simulink model "Dyn_Sim"  (Simulink 8.9)
settings: Solver=VariableStepAuto  StartTime=0.0  StopTime=time  FixedStep=0.1  MaxStep=0.1  RelTol=1e-3  EnableMultiTasking=on
values from neighbouring files (symbols this model uses):
  l1d = 2    [runner_simulation.m]
  l2d = 2    [runner_simulation.m]
  q0 = [gg gg 1]'.*[5 -4 pi/2]'    [runner_simulation.m]
  q0_1 = [gg gg 1]'.*[4 -6 pi/2]'    [runner_simulation.m]
  q0_2 = [gg gg 1]'.*[5 -6 pi/3]'    [runner_simulation.m]
  sai1_d = pi/2    (= 1.57079632679)    [runner_simulation.m]
  sai2_d = -pi/2    (= -1.57079632679)    [runner_simulation.m]
  u0 = [0.1;0.1;0.1]'    [runner_simulation.m]
  u01 = [0;0;0]'    [runner_simulation.m]
Description:
  | Real-Time Van der Pol Simulation
  | 
  | This demonstration shows a real-time version of the Simulink(R) Van der Pol
  | simulation demo. This model does not need any external signals, so it does
  | not need any data acquisition hardware or driver. This makes the model ideal
  | for first experiments with Real-Time Windows Target(TM), without need to
  | worry about proper I/O hardware configuration.
  | 
  | How to run this demo in Normal Mode:
  | 
  | 1) Double-click the orange button to switch to Normal Mode if needed.
  | 2) Start the real-time execution using Simulation->Start.
  | 3) Observe any missed ticks on the Missed Ticks scope.
  | 
  | How to run this demo in External Mode:
  | 
  | 1) Double-click the orange button to switch to External Mode if needed.
  | 2) Build the model using Tools->Code Generation->Build Model.
  | 3) Connect to the real-time code using Simulation->Connect to target.
  | 4) Start the real-time execution using Simulation->Start real-time code.
  | 5) Missed ticks will be always zero.
settings Model: Creator=The MathWorks Inc.  LastModifiedBy=Rasoul  ExtModeTrigDuration=101
settings DataIOCC: SignalLoggingSaveFormat=Dataset  SignalLoggingName=logsOut
settings OptimizationCC: ExpressionDepthLimit=2147483647  InitFltsAndDblsToZero=on  EfficientMapNaN2IntZero=off
settings DebuggingCC: SignalResolutionControl=TryResolveAllWithWarning  AllowSymbolicDim=off
settings HardwareCC: ProdBitPerPointer=64  ProdBitPerSizeT=64  ProdBitPerPtrDiffT=64  ProdLargestAtomicFloat=Float  ProdIntDivRoundTo=Zero  ProdEndianess=LittleEndian  ProdWordSize=64  ProdHWDeviceType=Intel->x86-64 (Windows64)  TargetBitPerLong=64  TargetBitPerPointer=64  TargetIntDivRoundTo=Zero  TargetEndianess=LittleEndian  TargetWordSize=64  TargetHWDeviceType=Intel->x86-64
settings RTWCC: SystemTargetFile=sldrt.tlc  TemplateMakefile=sldrt.tmf  Description=Simulink Desktop Real-Time  RTWCompilerOptimization=on
settings CodeAppCC: MaxIdLength=95
settings SimulinkDesktopRealTimeCC: TargetPreCompLibLocation=C:\Program Files\MATLAB\R2017a\toolbox\sldrt\lib\win64  TargetLangStandard=C89/C90 (ANSI)  SupportVariableSizeSignals=off

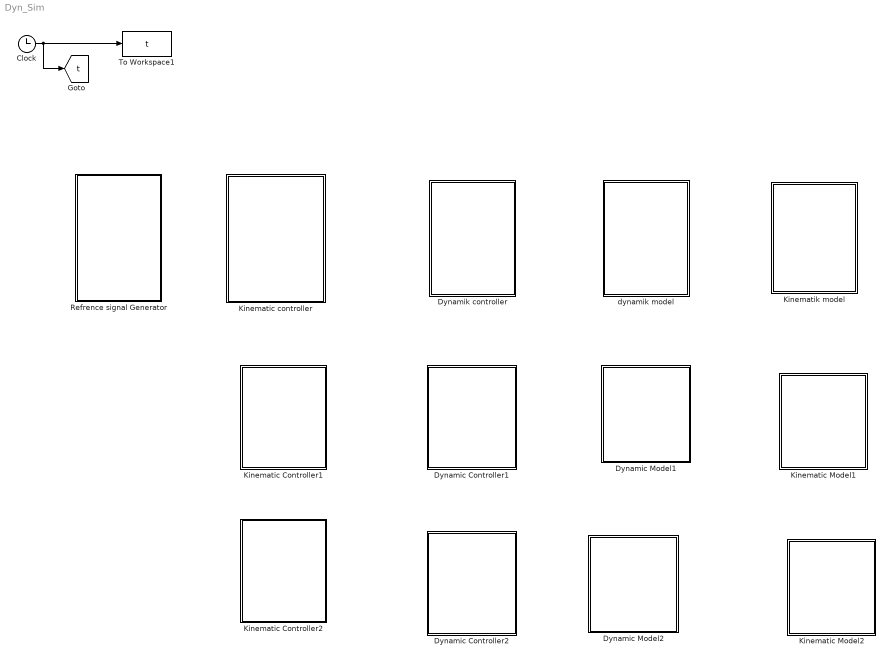
== system Dyn_Sim ==
  Clock : Clock
  Dynamic Controller1 : Subsystem
  Dynamic Controller2 : Subsystem
  Dynamic Model1 : Subsystem
  Dynamic Model2 : Subsystem
  Dynamik controller : Subsystem
  Kinematic Controller1 : Subsystem
  Kinematic Controller2 : Subsystem
  Kinematic Model1 : Subsystem
  Kinematic Model2 : Subsystem
  Kinematic controller : Subsystem
  Kinematik model : Subsystem
  "Refrence signal Generator " : Subsystem
  To Workspace1 : ToWorkspace  VariableName=t  SampleTime=-1
  dynamik model : Subsystem
  tag scope: t=global
  wires:
  Clock/1 -> To Workspace1/1, [t]

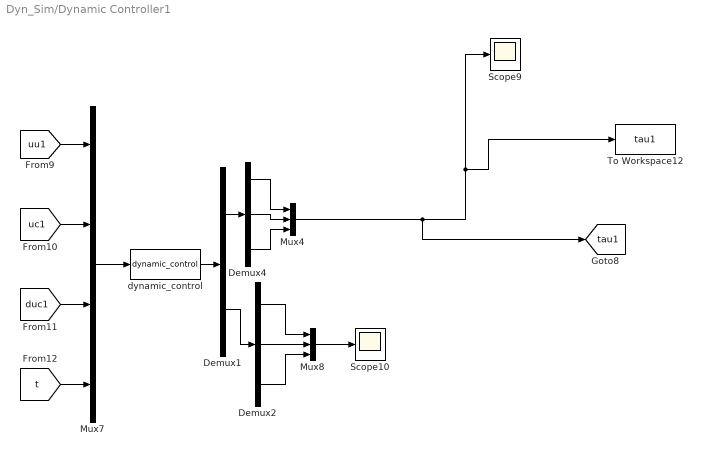
== system Dyn_Sim/Dynamic Controller1 ==
  Demux1 : Demux  Outputs=2
  Demux2 : Demux  Outputs=3
  Demux4 : Demux  Outputs=3
  Mux4 : Mux  Inputs=3
  Mux7 : Mux
  Mux8 : Mux  Inputs=3
  Scope10 : Scope
  Scope9 : Scope
  To Workspace12 : ToWorkspace  VariableName=tau1  SampleTime=-1
  dynamic_control : MATLABFcn  MATLABFcn=dynamic_control  OutputDimensions=6  OutputSignalType=real
  tag scope: tau1=global
  wires:
  Mux7/1 -> dynamic_control/1
  [duc1] -> Mux7/3
  Mux8/1 -> Scope10/1
  Demux4/1 -> Mux4/1
  [t] -> Mux7/4
  [uu1] -> Mux7/1
  [uc1] -> Mux7/2
  dynamic_control/1 -> Demux1/1
  Demux4/2 -> Mux4/2
  Demux1/1 -> Demux4/1
  Demux1/2 -> Demux2/1
  Demux2/1 -> Mux8/1
  Demux2/2 -> Mux8/2
  Demux4/3 -> Mux4/3
  Demux2/3 -> Mux8/3
  Mux4/1 -> Scope9/1, To Workspace12/1, [tau1]

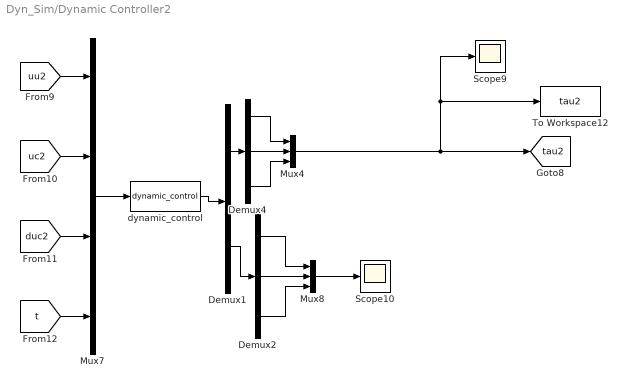
== system Dyn_Sim/Dynamic Controller2 ==
  Demux1 : Demux  Outputs=2
  Demux2 : Demux  Outputs=3
  Demux4 : Demux  Outputs=3
  Mux4 : Mux  Inputs=3
  Mux7 : Mux
  Mux8 : Mux  Inputs=3
  Scope10 : Scope
  Scope9 : Scope
  To Workspace12 : ToWorkspace  VariableName=tau2  SampleTime=-1
  dynamic_control : MATLABFcn  MATLABFcn=dynamic_control  OutputDimensions=6  OutputSignalType=real
  tag scope: tau2=global
  wires:
  Demux2/3 -> Mux8/3
  Demux4/3 -> Mux4/3
  Demux2/1 -> Mux8/1
  Demux4/1 -> Mux4/1
  Mux8/1 -> Scope10/1
  Demux2/2 -> Mux8/2
  [duc2] -> Mux7/3
  dynamic_control/1 -> Demux1/1
  [t] -> Mux7/4
  Demux1/2 -> Demux2/1
  Demux4/2 -> Mux4/2
  [uu2] -> Mux7/1
  Demux1/1 -> Demux4/1
  Mux7/1 -> dynamic_control/1
  [uc2] -> Mux7/2
  Mux4/1 -> [tau2], To Workspace12/1, Scope9/1

== system Dyn_Sim/Dynamic Model1 ==
  Integrator2 : Integrator  InitialCondition=u01
  Mux9 : Mux  Inputs=3
  To Workspace11 : ToWorkspace  VariableName=uu1  SampleTime=-1
  dynamic_model : MATLABFcn  MATLABFcn=dynamic_model  OutputDimensions=3  OutputSignalType=real
  tag scope: uu1=global
  wires:
  [tau1] -> Mux9/2
  [uu1] -> Mux9/1
  dynamic_model/1 -> Integrator2/1
  Mux9/1 -> dynamic_model/1
  [t] -> Mux9/3
  Integrator2/1 -> [uu1], To Workspace11/1

== system Dyn_Sim/Dynamic Model2 ==
  Integrator2 : Integrator  InitialCondition=u01
  Mux9 : Mux  Inputs=3
  To Workspace11 : ToWorkspace  VariableName=uu2  SampleTime=-1
  dynamic_model : MATLABFcn  MATLABFcn=dynamic_model  OutputDimensions=3  OutputSignalType=real
  tag scope: uu2=global
  wires:
  Mux9/1 -> dynamic_model/1
  [tau2] -> Mux9/2
  dynamic_model/1 -> Integrator2/1
  Integrator2/1 -> To Workspace11/1, [uu2]
  [t] -> Mux9/3
  [uu2] -> Mux9/1

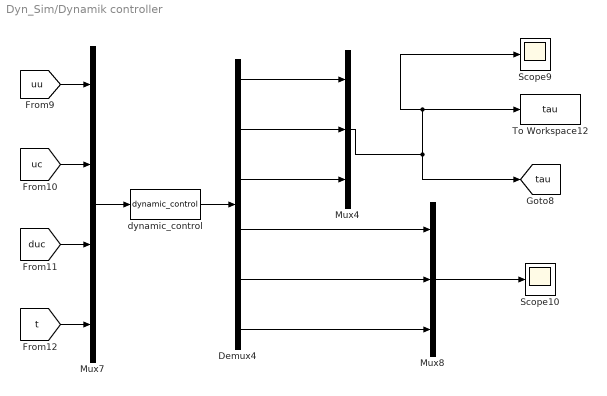
== system Dyn_Sim/Dynamik controller ==
  Demux4 : Demux  Outputs=6
  Mux4 : Mux  Inputs=3
  Mux7 : Mux
  Mux8 : Mux  Inputs=3
  Scope10 : Scope
  Scope9 : Scope
  To Workspace12 : ToWorkspace  VariableName=tau  SampleTime=-1
  dynamic_control : MATLABFcn  MATLABFcn=dynamic_control  OutputDimensions=6  OutputSignalType=real
  tag scope: tau=global
  wires:
  Demux4/6 -> Mux8/3
  Demux4/5 -> Mux8/2
  Demux4/3 -> Mux4/3
  dynamic_control/1 -> Demux4/1
  [uu] -> Mux7/1
  Mux8/1 -> Scope10/1
  Demux4/4 -> Mux8/1
  [duc] -> Mux7/3
  [uc] -> Mux7/2
  Demux4/1 -> Mux4/1
  Demux4/2 -> Mux4/2
  Mux7/1 -> dynamic_control/1
  [t] -> Mux7/4
  Mux4/1 -> [tau], Scope9/1, To Workspace12/1

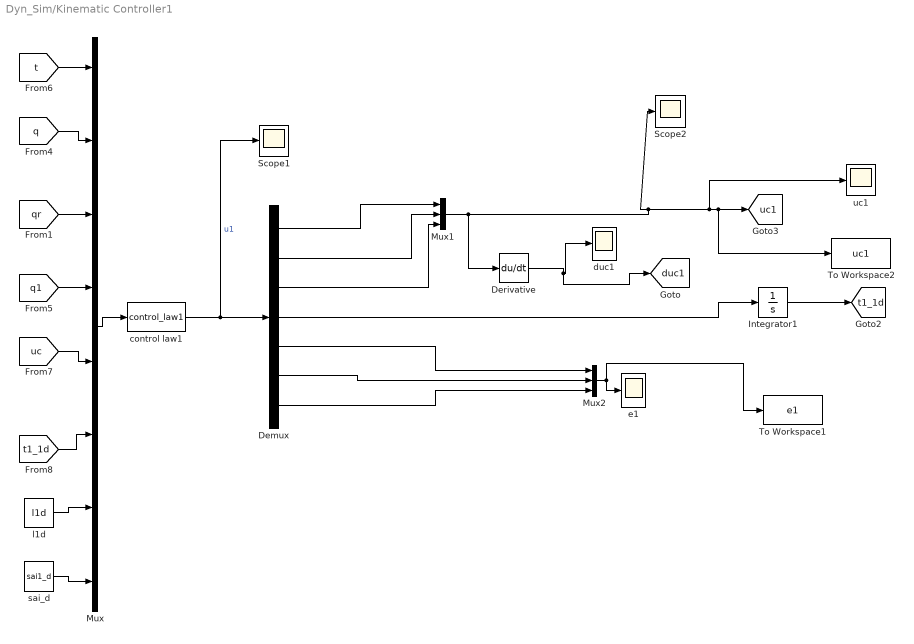
== system Dyn_Sim/Kinematic Controller1 ==
  Demux : Demux  Outputs=7
  Derivative : Derivative
  Integrator1 : Integrator  InitialCondition=pi/2
  Mux : Mux  Inputs=8
  Mux1 : Mux  Inputs=3
  Mux2 : Mux  Inputs=3
  Scope1 : Scope
  Scope2 : Scope
  To Workspace1 : ToWorkspace  VariableName=e1  SampleTime=-1
  To Workspace2 : ToWorkspace  VariableName=uc1  SampleTime=-1
  control law1 : MATLABFcn  MATLABFcn=control_law1  OutputDimensions=7  OutputSignalType=real
  duc1 : Scope
  e1 : Scope
  l1d : Constant  Value=l1d
  sai_d : Constant  Value=sai1_d
  uc1 : Scope
  tag scope: duc1=global, t1_1d=global, uc1=global
  wires:
  control law1/1 -> Scope1/1, Demux/1  "u1"
  Mux/1 -> control law1/1
  Integrator1/1 -> [t1_1d]
  Mux1/1 -> Derivative/1, uc1/1, To Workspace2/1, [uc1], Scope2/1
  Demux/1 -> Mux1/1
  Demux/2 -> Mux1/2
  Mux2/1 -> e1/1, To Workspace1/1
  Derivative/1 -> [duc1], duc1/1
  [uc] -> Mux/5
  [q1] -> Mux/4
  [qr] -> Mux/3
  [q] -> Mux/2
  [t] -> Mux/1
  [t1_1d] -> Mux/6
  l1d/1 -> Mux/7
  sai_d/1 -> Mux/8
  Demux/3 -> Mux1/3
  Demux/4 -> Integrator1/1
  Demux/5 -> Mux2/1
  Demux/6 -> Mux2/2
  Demux/7 -> Mux2/3

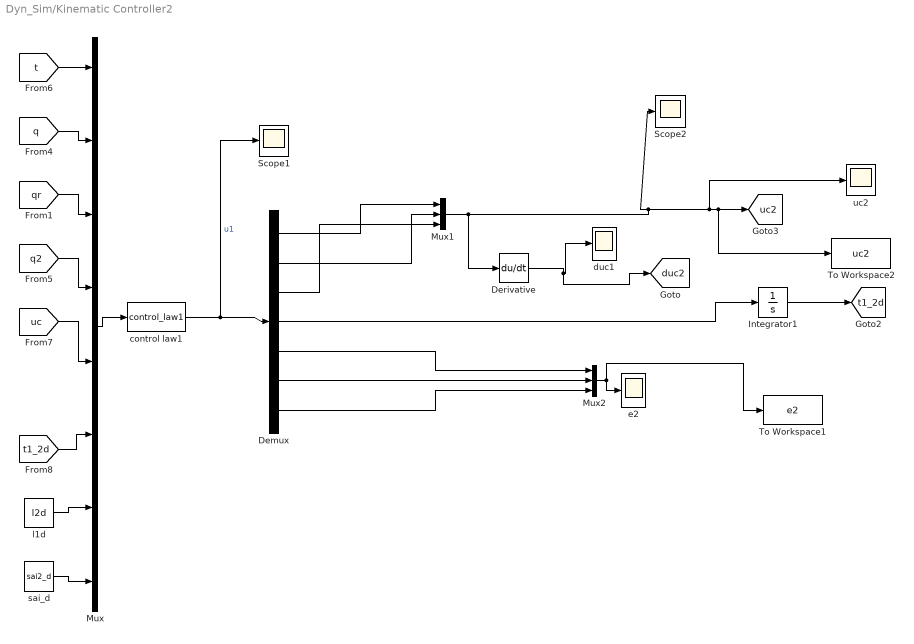
== system Dyn_Sim/Kinematic Controller2 ==
  Demux : Demux  Outputs=7
  Derivative : Derivative
  Integrator1 : Integrator  InitialCondition=pi/2
  Mux : Mux  Inputs=8
  Mux1 : Mux  Inputs=3
  Mux2 : Mux  Inputs=3
  Scope1 : Scope
  Scope2 : Scope
  To Workspace1 : ToWorkspace  VariableName=e2  SampleTime=-1
  To Workspace2 : ToWorkspace  VariableName=uc2  SampleTime=-1
  control law1 : MATLABFcn  MATLABFcn=control_law1  OutputDimensions=7  OutputSignalType=real
  duc1 : Scope
  e2 : Scope
  l1d : Constant  Value=l2d
  sai_d : Constant  Value=sai2_d
  uc2 : Scope
  tag scope: duc2=global, t1_2d=global, uc2=global
  wires:
  Mux/1 -> control law1/1
  control law1/1 -> Demux/1, Scope1/1  "u1"
  Mux1/1 -> Scope2/1, [uc2], To Workspace2/1, uc2/1, Derivative/1
  Integrator1/1 -> [t1_2d]
  Demux/1 -> Mux1/1
  [q2] -> Mux/4
  Demux/2 -> Mux1/2
  Derivative/1 -> duc1/1, [duc2]
  [t] -> Mux/1
  [uc] -> Mux/5
  [qr] -> Mux/3
  [q] -> Mux/2
  Mux2/1 -> To Workspace1/1, e2/1
  [t1_2d] -> Mux/6
  l1d/1 -> Mux/7
  sai_d/1 -> Mux/8
  Demux/3 -> Mux1/3
  Demux/4 -> Integrator1/1
  Demux/5 -> Mux2/1
  Demux/6 -> Mux2/2
  Demux/7 -> Mux2/3

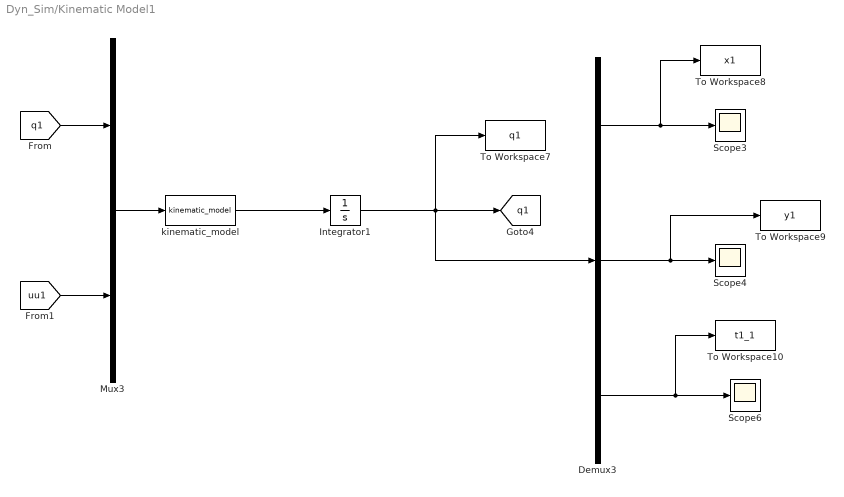
== system Dyn_Sim/Kinematic Model1 ==
  Demux3 : Demux  Outputs=3
  Integrator1 : Integrator  InitialCondition=q0_1
  Mux3 : Mux  Inputs=2
  Scope3 : Scope
  Scope4 : Scope
  Scope6 : Scope
  To Workspace10 : ToWorkspace  VariableName=t1_1  SampleTime=-1
  To Workspace7 : ToWorkspace  VariableName=q1  SampleTime=-1
  To Workspace8 : ToWorkspace  VariableName=x1  SampleTime=-1
  To Workspace9 : ToWorkspace  VariableName=y1  SampleTime=-1
  kinematic_model : MATLABFcn  MATLABFcn=kinematic_model  OutputDimensions=3  OutputSignalType=real
  tag scope: q1=global
  wires:
  [q1] -> Mux3/1
  [uu1] -> Mux3/2
  Mux3/1 -> kinematic_model/1
  Demux3/3 -> Scope6/1, To Workspace10/1
  Demux3/1 -> Scope3/1, To Workspace8/1
  Demux3/2 -> Scope4/1, To Workspace9/1
  kinematic_model/1 -> Integrator1/1
  Integrator1/1 -> [q1], Demux3/1, To Workspace7/1

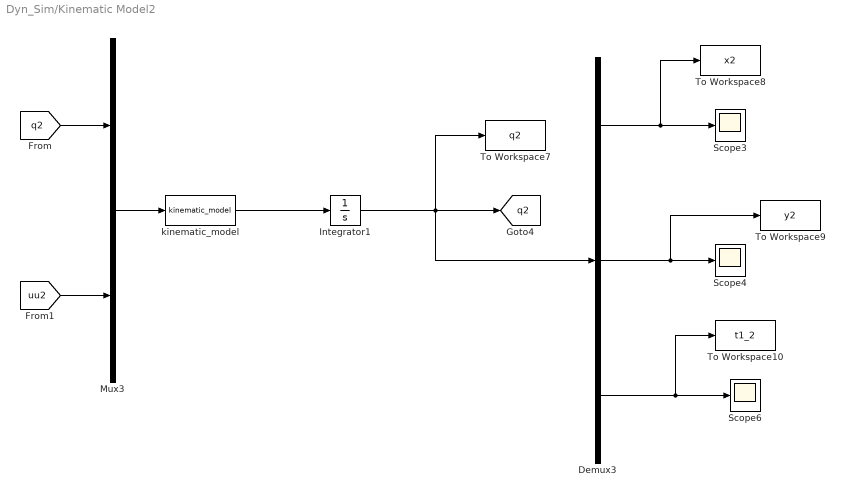
== system Dyn_Sim/Kinematic Model2 ==
  Demux3 : Demux  Outputs=3
  Integrator1 : Integrator  InitialCondition=q0_2
  Mux3 : Mux  Inputs=2
  Scope3 : Scope
  Scope4 : Scope
  Scope6 : Scope
  To Workspace10 : ToWorkspace  VariableName=t1_2  SampleTime=-1
  To Workspace7 : ToWorkspace  VariableName=q2  SampleTime=-1
  To Workspace8 : ToWorkspace  VariableName=x2  SampleTime=-1
  To Workspace9 : ToWorkspace  VariableName=y2  SampleTime=-1
  kinematic_model : MATLABFcn  MATLABFcn=kinematic_model  OutputDimensions=3  OutputSignalType=real
  tag scope: q2=global
  wires:
  Mux3/1 -> kinematic_model/1
  Demux3/2 -> To Workspace9/1, Scope4/1
  Demux3/1 -> To Workspace8/1, Scope3/1
  [q2] -> Mux3/1
  [uu2] -> Mux3/2
  kinematic_model/1 -> Integrator1/1
  Demux3/3 -> To Workspace10/1, Scope6/1
  Integrator1/1 -> To Workspace7/1, Demux3/1, [q2]

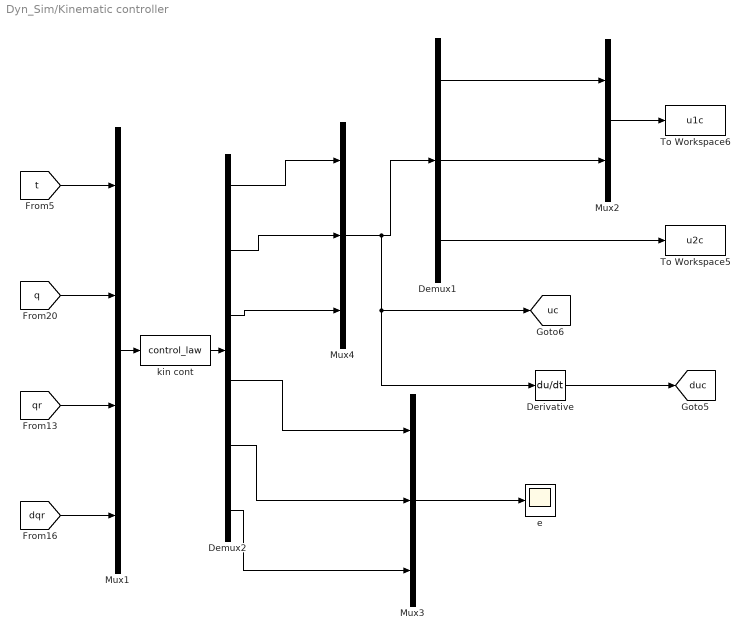
== system Dyn_Sim/Kinematic controller ==
  Demux1 : Demux  Outputs=3
  Demux2 : Demux  Outputs=6
  Derivative : Derivative
  Mux1 : Mux
  Mux2 : Mux  Inputs=2
  Mux3 : Mux  Inputs=3
  Mux4 : Mux  Inputs=3
  To Workspace5 : ToWorkspace  VariableName=u2c  SampleTime=-1
  To Workspace6 : ToWorkspace  VariableName=u1c  SampleTime=-1
  e : Scope
  kin cont : MATLABFcn  MATLABFcn=control_law  OutputDimensions=6  OutputSignalType=real
  tag scope: duc=global, uc=global
  wires:
  kin cont/1 -> Demux2/1
  Mux1/1 -> kin cont/1
  [t] -> Mux1/1
  Derivative/1 -> [duc]
  [qr] -> Mux1/3
  [q] -> Mux1/2
  [dqr] -> Mux1/4
  Demux1/3 -> To Workspace5/1
  Demux1/2 -> Mux2/2
  Demux1/1 -> Mux2/1
  Mux2/1 -> To Workspace6/1
  Demux2/4 -> Mux3/1
  Demux2/5 -> Mux3/2
  Demux2/6 -> Mux3/3
  Mux3/1 -> e/1
  Demux2/1 -> Mux4/1
  Demux2/2 -> Mux4/2
  Demux2/3 -> Mux4/3
  Mux4/1 -> Derivative/1, [uc], Demux1/1

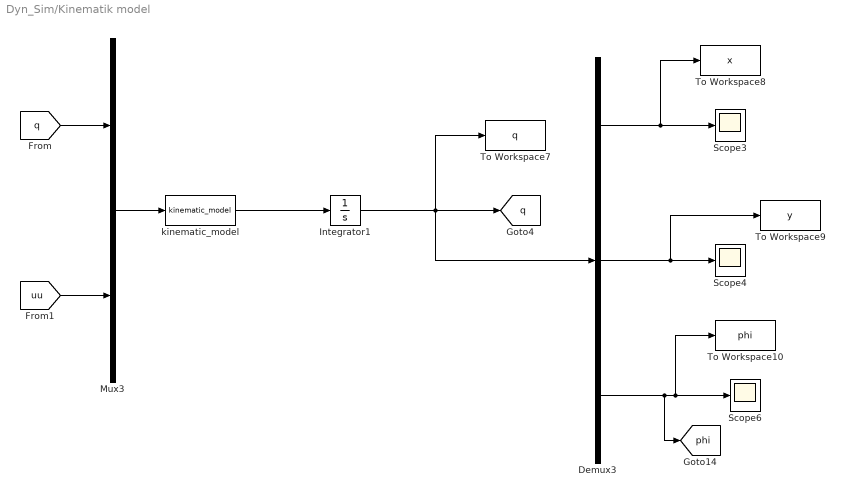
== system Dyn_Sim/Kinematik model ==
  Demux3 : Demux  Outputs=3
  Integrator1 : Integrator  InitialCondition=q0
  Mux3 : Mux  Inputs=2
  Scope3 : Scope
  Scope4 : Scope
  Scope6 : Scope
  To Workspace10 : ToWorkspace  VariableName=phi  SampleTime=-1
  To Workspace7 : ToWorkspace  VariableName=q  SampleTime=-1
  To Workspace8 : ToWorkspace  VariableName=x  SampleTime=-1
  To Workspace9 : ToWorkspace  VariableName=y  SampleTime=-1
  kinematic_model : MATLABFcn  MATLABFcn=kinematic_model  OutputDimensions=3  OutputSignalType=real
  tag scope: phi=global, q=global
  wires:
  Integrator1/1 -> [q], Demux3/1, To Workspace7/1
  Demux3/2 -> Scope4/1, To Workspace9/1
  kinematic_model/1 -> Integrator1/1
  Demux3/3 -> [phi], Scope6/1, To Workspace10/1
  [uu] -> Mux3/2
  Mux3/1 -> kinematic_model/1
  [q] -> Mux3/1
  Demux3/1 -> Scope3/1, To Workspace8/1

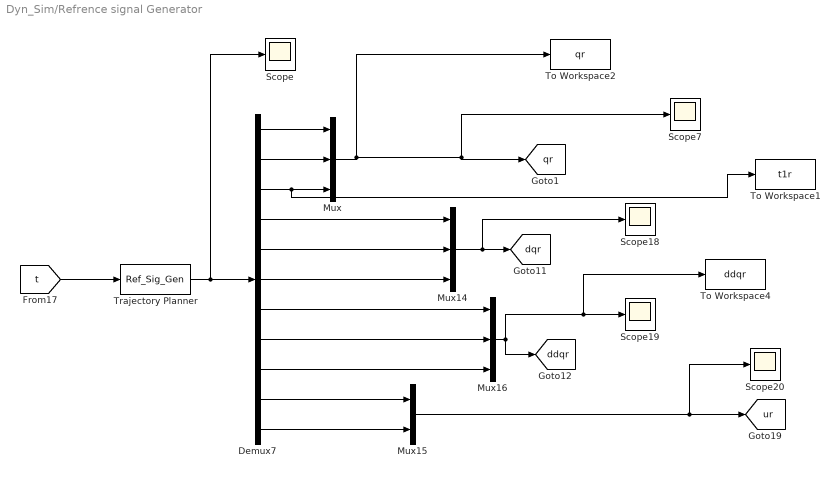
== system Dyn_Sim/Refrence signal Generator  ==
  Demux7 : Demux  Outputs=11
  Mux : Mux  Inputs=3
  Mux14 : Mux  Inputs=3
  Mux15 : Mux  Inputs=2
  Mux16 : Mux  Inputs=3
  Scope{,7,18..20} (5 alike) : Scope
  To Workspace1 : ToWorkspace  VariableName=t1r  SampleTime=-1
      settings: Save2DSignal=2-D array (concatenate along first dimension)
  To Workspace2 : ToWorkspace  VariableName=qr  SampleTime=-1
      settings: Save2DSignal=2-D array (concatenate along first dimension)
  To Workspace4 : ToWorkspace  VariableName=ddqr  SampleTime=-1
      settings: Save2DSignal=2-D array (concatenate along first dimension)
  Trajectory Planner : MATLABFcn  MATLABFcn=Ref_Sig_Gen  OutputDimensions=11
  tag scope: ddqr=global, dqr=global, qr=global, ur=global
  wires:
  Trajectory Planner/1 -> Scope/1, Demux7/1
  Demux7/1 -> Mux/1
  [t] -> Trajectory Planner/1
  Demux7/9 -> Mux16/3
  Demux7/6 -> Mux14/3
  Mux15/1 -> Scope20/1, [ur]
  Demux7/5 -> Mux14/2
  Demux7/10 -> Mux15/1
  Demux7/2 -> Mux/2
  Demux7/3 -> To Workspace1/1, Mux/3
  Mux16/1 -> [ddqr], To Workspace4/1, Scope19/1
  Demux7/7 -> Mux16/1
  Mux/1 -> To Workspace2/1, Scope7/1, [qr]
  Demux7/11 -> Mux15/2
  Mux14/1 -> Scope18/1, [dqr]
  Demux7/4 -> Mux14/1
  Demux7/8 -> Mux16/2

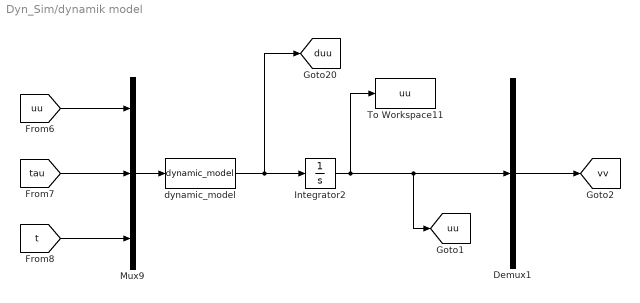
== system Dyn_Sim/dynamik model ==
  Demux1 : Demux  Outputs=3
  Integrator2 : Integrator  InitialCondition=u0
  Mux9 : Mux  Inputs=3
  To Workspace11 : ToWorkspace  VariableName=uu  SampleTime=-1
  dynamic_model : MATLABFcn  MATLABFcn=dynamic_model  OutputDimensions=3  OutputSignalType=real
  tag scope: duu=global, uu=global, vv=global
  wires:
  Demux1/2 -> [vv]
  Integrator2/1 -> To Workspace11/1, Demux1/1, [uu]
  [uu] -> Mux9/1
  [t] -> Mux9/3
  Mux9/1 -> dynamic_model/1
  dynamic_model/1 -> Integrator2/1, [duu]
  [tau] -> Mux9/2
